simulink subsystem "StreetLaneSegment2x2_asSubsystem"  (R2021a)
settings: Solver=VariableStepAuto  StartTime=0.0  StopTime=10.0  RelTol=1e-3
settings Model: Creator=phill  LastModifiedBy=phill

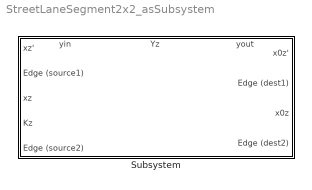
== system StreetLaneSegment2x2_asSubsystem ==
  Subsystem : Subsystem  mask{Kz=0, Tz=0}
      mask prompts: Kz "Kz (Capacity - How many cars fit into this cell)"; Tz "Tz (Nominal travel time for vehicles traveling unobstructed through the cell)"
      mask help: The 2x2 extension to the basic cell.
      settings: PortSchema="{\"entries\":[{\"content\":{\"sides\":[{\"content\":{\"connectorIds\":[\"Out6\",\"In1\",\"Out7\",\"Out8\",\"In2\"]},\"type\":\"ConnectorPlacement.EquallySpacedRectSide\",\"uuid\":\"25df2790-c866-41ff-9dfe-266b31cf62ba\"},{\"content\":{\"connectorIds\":[\"Out1\",\"In3\",\"Out2\",\"In4\"],\"side\":\"RIGHT\"},\"type\":\"ConnectorPlacement.EquallySpacedRectSide\",\"uuid\":\"25d72334-2b21-4272-a907-00400a727cc8\"},{\"content\":{\"connectorIds\":[\"Out3\",\"Out4\",\"Out5\"],\"side\":\"TOP\"},\"type\":\"ConnectorPlacement.EquallySpacedRectSide\",\"uuid\":\"016a1f1d-ac45-4b29-877f-ff17231147ed\"}]},\"type\":\"ConnectorPlacement.EquallySpacedConnector\",\"uuid\":\"d9a39936-9630-4e37-953d-f1129270bc17\"}],\"packageUris\":[\"http://schema.mathworks.com/mf0/Connector/R2020b\"],\"version\":\"1.0\"}"
      mask Display:
      | image('$imagefile'); % Use "Edit Image" on toolstrip to change.
      | %image('.\LaneIconLightGrey.png');
      | disp('Street Lane Segment 2x2 \n\n');
      | disp(['Kz = ', get_param(gcb,'Kz'), ' | Tz = ', get_param(gcb, 'Tz')])

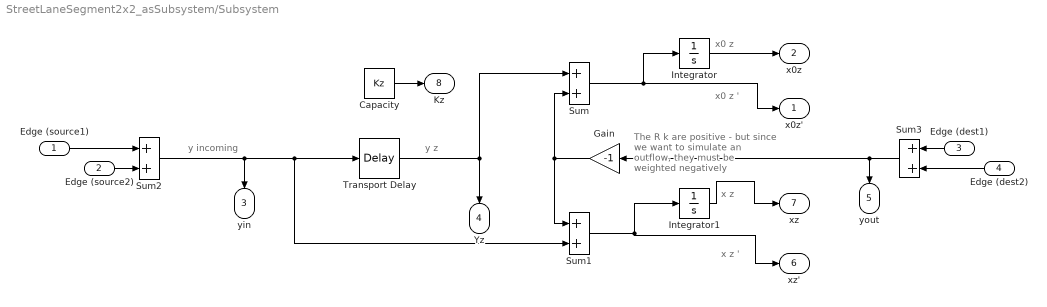
== system StreetLaneSegment2x2_asSubsystem/Subsystem ==
  note: x z
  note: x0 z
  note: x z '
  note: x0 z '
  note: y incoming
  note: The R k are positive - but since we
      | want to simulate an outflow, they
      | must be weighted negatively
  note: y z
  Edge (source1) : Inport
  Edge (source2) : Inport  Port=2
  Edge (dest1) : Inport  Port=3
  Edge (dest2) : Inport  Port=4
  Capacity : Constant  Value=Kz
  Gain : Gain  Gain=-1
  Integrator : Integrator
  Integrator1 : Integrator
  Sum{,1..3} (4 alike) : Sum
  Transport Delay : TransportDelay  DelayTime=Tz
  x0z' : Outport
  x0z : Outport  Port=2
  yin : Outport  Port=3
  Yz : Outport  Port=4
  yout : Outport  Port=5
  xz' : Outport  Port=6
  xz : Outport  Port=7
  Kz : Outport  Port=8
  wires:
  Integrator/1 -> x0z/1
  Transport Delay/1 -> Yz/1, Sum/1
  Sum1/1 -> xz'/1, Integrator1/1
  Edge (source2)/1 -> Sum2/2
  Edge (source1)/1 -> Sum2/1
  Capacity/1 -> Kz/1
  Sum2/1 -> yin/1, Sum1/2, Transport Delay/1
  Sum3/1 -> yout/1, Gain/1
  Edge (dest2)/1 -> Sum3/2
  Sum/1 -> x0z'/1, Integrator/1
  Gain/1 -> Sum1/1, Sum/2
  Edge (dest1)/1 -> Sum3/1
  Integrator1/1 -> xz/1
